simulink model "pv1"  (Simulink 6.5)
settings: Solver=VariableStepDiscrete  StartTime=0.0  StopTime=1  MaxStep=0.02  RelTol=1e-3
libraries: simulink x3
settings Model: Creator=Mama  LastModifiedBy=Dragan Maksimovic
settings DebuggingCC: AlgebraicLoopMsg=none  SolverPrmCheckMsg=none  UnconnectedOutputMsg=none

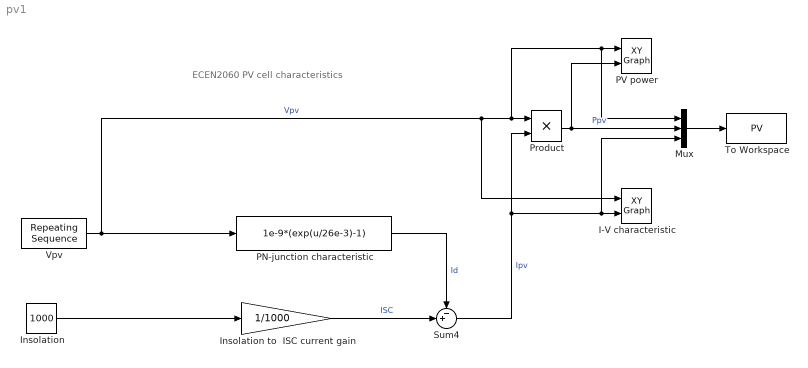
== system pv1 ==
  note: ECEN2060
      | PV cell characteristics
  I-V characteristic : simulink/Sinks/XY Graph  SystemSampleTime=-1  xmin=0  xmax=0.6  ymin=0  ymax=1  st=-1
  Insolation : Constant  Value=1000  OutDataType=sfix(16)  ConRadixGroup=Use specified scaling  OutScaling=2^0  SampleTime=inf  FramePeriod=inf
  Insolation to  ISC current gain : Gain  Gain=1/1000
  Mux : Mux  Inputs=3
  PN-junction characteristic : Fcn  Expr=1e-9*(exp(u/26e-3)-1)
  PV power : simulink/Sinks/XY Graph  SystemSampleTime=-1  xmin=0  xmax=0.6  ymin=0  ymax=0.5  st=-1
  Product : Product  RndMeth=Zero
  Sum4 : Sum  Inputs=-+|
  To Workspace : ToWorkspace  VariableName=PV  SampleTime=-1  SaveFormat=Structure With Time
  Vpv : simulink/Sources/Repeating Sequence  SystemSampleTime=-1  rep_seq_t=[0 1 2]  rep_seq_y=[-0.1 0.6 -0.1]
  wires:
  Insolation to  ISC current gain/1 -> Sum4/2  "ISC"
  PN-junction characteristic/1 -> Sum4/1  "Id"
  Insolation/1 -> Insolation to  ISC current gain/1
  Sum4/1 -> Product/2, I-V characteristic/2, Mux/3  "Ipv"
  Product/1 -> PV power/2, Mux/2  "Ppv"
  Vpv/1 -> Product/1, PV power/1, Mux/1, I-V characteristic/1, PN-junction characteristic/1  "Vpv"
  Mux/1 -> To Workspace/1
